simulink model "Question_3"  (R2024b)
settings: Solver=VariableStepAuto  StartTime=0.0  StopTime=10.0  RelTol=1e-3
model workspace (MAT data in the model file):
  B = 100
  K1 = 100
  K12 = 100
  M1 = 200
  M2 = 2000
undefined symbols (not defined in the file): y1, y2
settings Model: Creator=Sagar  LastModifiedBy=Sagar

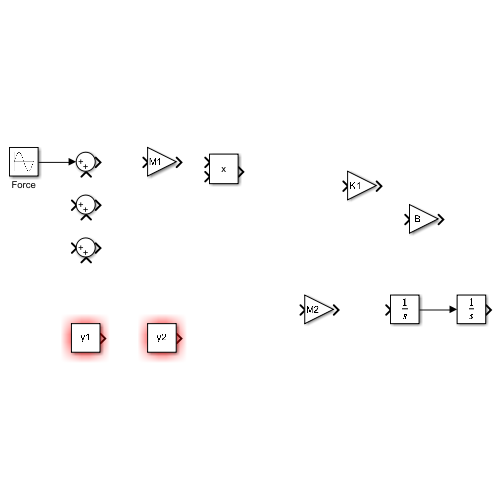
[thumbnail: Simulink's stored preview of the top-level diagram]
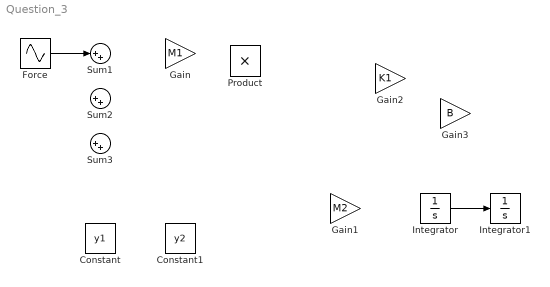
== system Question_3 ==
  Constant : Constant  Value=y1
  Constant1 : Constant  Value=y2
  Force : Sin  SampleTime=0
  Gain : Gain  Gain=M1
  Gain1 : Gain  Gain=M2
  Gain2 : Gain  Gain=K1
  Gain3 : Gain  Gain=B
  Integrator : Integrator
  Integrator1 : Integrator
  Product : Product
  Sum1 : Sum  Inputs=|++
  Sum2 : Sum  Inputs=|++
  Sum3 : Sum  Inputs=|++
  wires:
  Integrator/1 -> Integrator1/1
  Force/1 -> Sum1/1
